simulink model "High_Pass_Filter"  (R2017a)
settings: Solver=FixedStepAuto  StartTime=0.0  StopTime=10.0  FixedStep=0.001  RelTol=1e-3
undefined symbols (not defined in the file or in its folder): DiscIntNeverNeededParam
settings Model: Creator=LocalAccount  LastModifiedBy=vivek_000

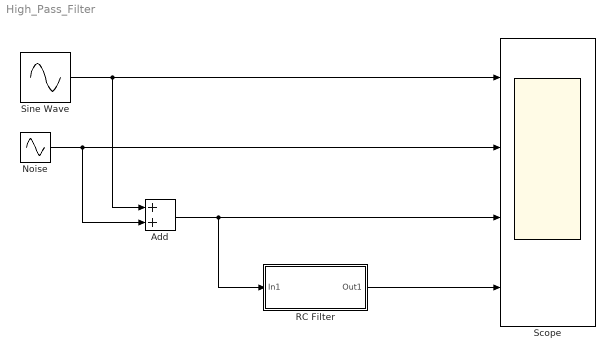
== system High_Pass_Filter ==
  Add : Sum
  Noise : Sin  Amplitude=10  Frequency=5  SampleTime=0
  RC Filter : Subsystem
  Scope : Scope  NumInputPorts=4
  Sine Wave : Sin  Amplitude=100  Frequency=100  SampleTime=0
  wires:
  Noise/1 -> Add/2, Scope/2
  Sine Wave/1 -> Add/1, Scope/1
  Add/1 -> RC Filter/1(In1), Scope/3
  RC Filter/1(Out1) -> Scope/4

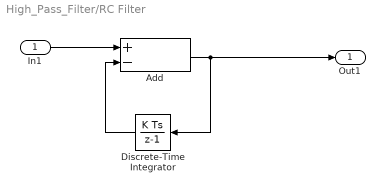
== system High_Pass_Filter/RC Filter ==
  In1 : Inport
  Add : Sum  Inputs=+-
  Discrete-Time Integrator : DiscreteIntegrator  gainval=100.0  InitialConditionSetting=State (most efficient)  SampleTime=-1  ICPrevOutput=DiscIntNeverNeededParam  ICPrevScaledInput=DiscIntNeverNeededParam
  Out1 : Outport
  wires:
  In1/1 -> Add/1
  Add/1 -> Discrete-Time Integrator/1, Out1/1
  Discrete-Time Integrator/1 -> Add/2
